simulink model "robustMPC_getInput_mdl"  (R2013a)
settings: Solver=ode45  StartTime=0.0  StopTime=10.0  RelTol=1e-3
undefined symbols (not defined in the file or in its folder): sol_x_mp
settings Model: Creator=Kostas  LastModifiedBy=Kostas

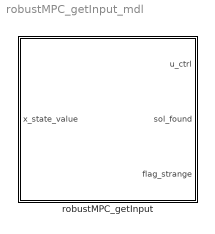
== system robustMPC_getInput_mdl ==
  robustMPC_getInput : Subsystem

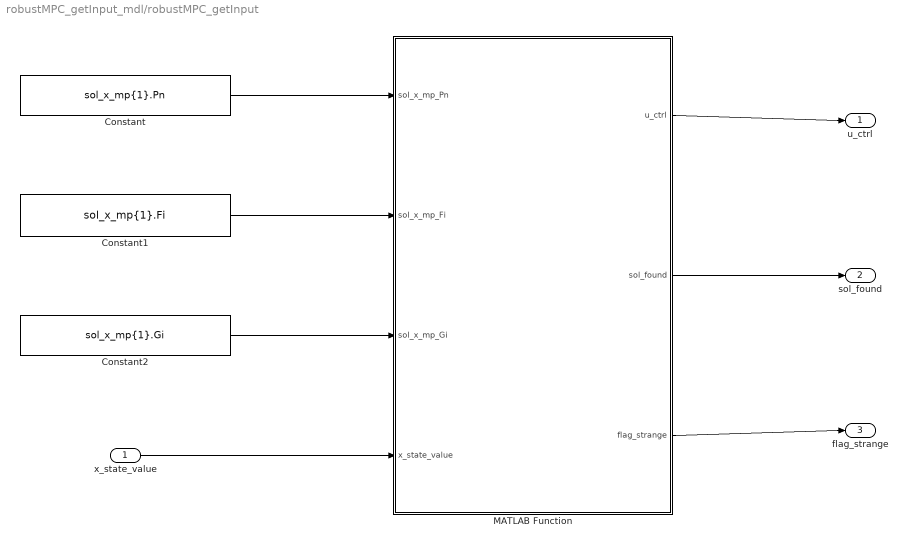
== system robustMPC_getInput_mdl/robustMPC_getInput ==
  x_state_value : Inport
  Constant : Constant  Value=sol_x_mp{1}.Pn
  Constant1 : Constant  Value=sol_x_mp{1}.Fi
  Constant2 : Constant  Value=sol_x_mp{1}.Gi
  MATLAB Function : MATLAB Function  TreatAsAtomicUnit=on
  u_ctrl : Outport
  sol_found : Outport  Port=2
  flag_strange : Outport  Port=3
  wires:
  Constant/1 -> MATLAB Function/1(sol_x_mp_Pn)
  Constant1/1 -> MATLAB Function/2(sol_x_mp_Fi)
  Constant2/1 -> MATLAB Function/3(sol_x_mp_Gi)
  x_state_value/1 -> MATLAB Function/4(x_state_value)
  MATLAB Function/1(u_ctrl) -> u_ctrl/1
  MATLAB Function/2(sol_found) -> sol_found/1
  MATLAB Function/3(flag_strange) -> flag_strange/1

== matlab function robustMPC_getInput_mdl/robustMPC_getInput/MATLAB Function ==
  data: sol_x_mp_Pn input; sol_x_mp_Fi input; sol_x_mp_Gi input; u_ctrl output; x_state_value input; sol_found output; flag_strange output
function [u_ctrl,sol_found, flag_strange] = robustmpc_getInput(sol_x_mp_Pn, sol_x_mp_Fi,sol_x_mp_Gi,x_state_value)
%
%   get control action from the explicit robust mpc computed using YALMIP
%
%   Syntax:
%   [u_ctrl,sol_found] = robustmpc_getInput(sol_x_mp, x_state_value)
%
%   Inputs:
%   sol_x_mp        : Multiparametric Robust MPC explicit solution
%   x_state_value   : value of the state vector
%
%   Outputs:
%   u_ctrl          : control action
%   sol_found       : flag indicating whether a solution was found
%
%   Authors: Kostas Alexis (konstantinos.alexis@mavt.ethz.ch)

sol_found = 1;
[i,j] = isinside(sol_x_mp_Pn, x_state_value);

flag_strange = 0;
if(length(j)>1)
    j = j(1); % this requires further analysis
    flag_strange = 1;
end

if(isempty(j)==0)
    u_ctrl = sol_x_mp_Fi{j}*x_state_value + sol_x_mp_Gi{j};
    sol_found = 1;
else
    sol_found = 0;
    u_ctrl = NaN;
end

if(flag_strange == 1)
    u_ctrl = 0.0256;
end
end
